simulink model "lag"  (R2019a)
settings: Solver=VariableStepAuto  StartTime=0.0  StopTime=10.0  RelTol=1e-3
settings Model: Creator=amah2  LastModifiedBy=amah2

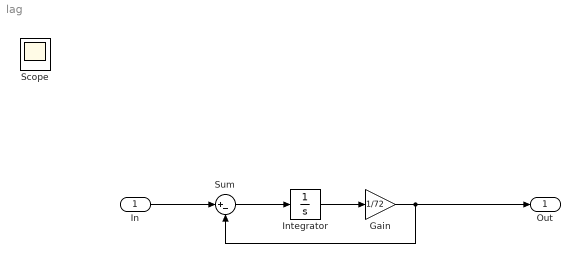
== system lag ==
  In : Inport
  Gain : Gain  Gain=1/72
  Integrator : Integrator
  Sum : Sum  Inputs=|+-
  Out : Outport
  Scope : Scope
  wires:
  Sum/1 -> Integrator/1
  In/1 -> Sum/1
  Gain/1 -> Sum/2, Out/1
  Integrator/1 -> Gain/1
